simulink model "Lightning_McSeas_Dashboard_Copy"  (R2021b)
settings: Solver=VariableStepAuto  StartTime=0.0  StopTime=inf  RelTol=1e-3
undefined symbols (not defined in the file): canChannel
libraries: canmsglib x15, canlib x11
(part 2 of 2)

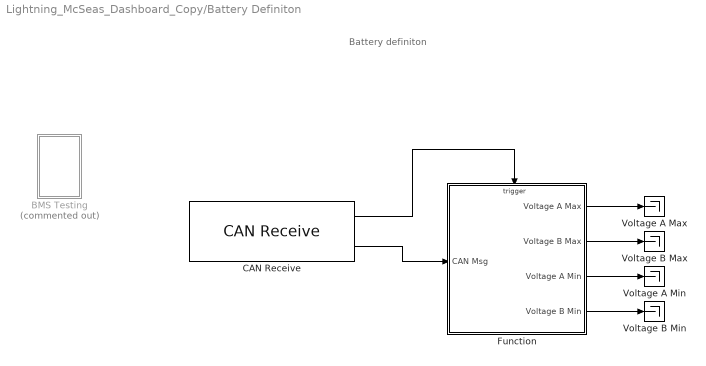
== system Lightning_McSeas_Dashboard_Copy/Battery Definiton ==
  note: Battery definiton
  BMS Testing : Subsystem  Commented=on
  CAN Receive : canlib/CAN Receive  BlockHandle=5.0006  Device=MathWorks Virtual 1 (Channel 1)  DeviceMenu=MathWorks Virtual 1 (Channel 1)  ObjConstructor=canChannel('MathWorks', 'Virtual 1', 1)  EnableStandardIDsFilter=off  StdIDsCombo=Allow all  StandardIDs=1536  EnableExtendedIDsFilter=off  ExtIDsCombo=Allow all  ExtendedIDs=0  SampleTime=0.1  MsgsPerTimestep=all  InternalFilterUpdateStatus=on  BusOutput=off
      settings: SourceProductBaseCode=VN
  Function : Subsystem  TreatAsAtomicUnit=on
  Voltage A Max : Terminator
  Voltage A Min : Terminator
  Voltage B Max : Terminator
  Voltage B Min : Terminator
  wires:
  CAN Receive/2 -> Function/1(CAN Msg)
  Function/1(Voltage A Max) -> Voltage A Max/1
  CAN Receive/1 -> Function/Trigger
  Function/2(Voltage B Max) -> Voltage B Max/1
  Function/3(Voltage A Min) -> Voltage A Min/1
  Function/4(Voltage B Min) -> Voltage B Min/1

== system Lightning_McSeas_Dashboard_Copy/GPS Definintion ==
  note: GPS definiton
  CAN Receive : canlib/CAN Receive  BlockHandle=24.0006  Device=MathWorks Virtual 1 (Channel 1)  DeviceMenu=MathWorks Virtual 1 (Channel 1)  ObjConstructor=canChannel('MathWorks', 'Virtual 1', 1)  EnableStandardIDsFilter=off  StdIDsCombo=Allow all  StandardIDs=1536  EnableExtendedIDsFilter=off  ExtIDsCombo=Allow all  ExtendedIDs=0  SampleTime=0.1  MsgsPerTimestep=all  InternalFilterUpdateStatus=on  BusOutput=off
      settings: SourceProductBaseCode=VN
  GPS Function : Subsystem  TreatAsAtomicUnit=on
  Speed : Terminator
  wires:
  CAN Receive/2 -> GPS Function/1(CAN Msg)
  GPS Function/1(Speed) -> Speed/1
  CAN Receive/1 -> GPS Function/Trigger

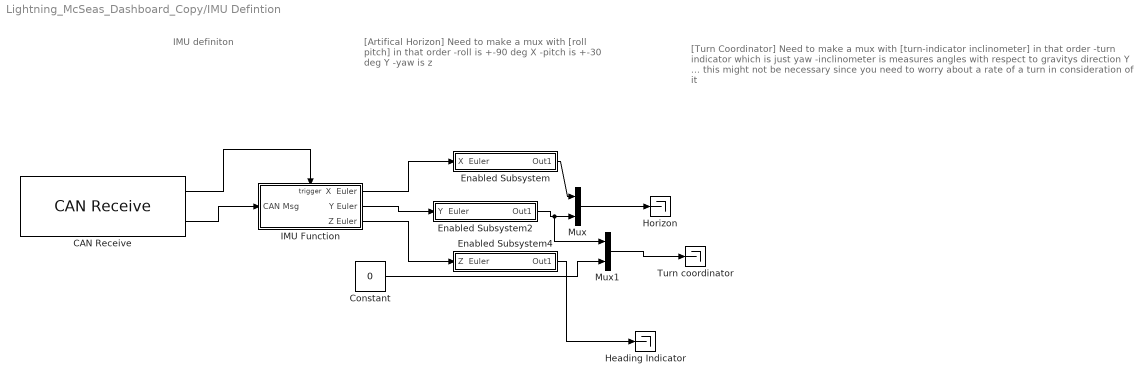
== system Lightning_McSeas_Dashboard_Copy/IMU Defintion ==
  note: [Turn Coordinator]
      | Need to make a mux with [turn-indicator inclinometer] in that order
      | -turn indicator which is just yaw
      |
      | -inclinometer is measures angles with respect to gravitys direction Y
      |
      | ... this might not be necessary since you need to worry about a rate of a turn in consideration of it
  note: [Artifical Horizon]
      | Need to make a mux with [roll pitch] in that order
      | -roll is +-90 deg X
      | -pitch is +-30 deg Y
      |
      | -yaw is z
  note: IMU definiton
  CAN Receive : canlib/CAN Receive  BlockHandle=40.0006  Device=MathWorks Virtual 1 (Channel 1)  DeviceMenu=MathWorks Virtual 1 (Channel 1)  ObjConstructor=canChannel('MathWorks', 'Virtual 1', 1)  EnableStandardIDsFilter=off  StdIDsCombo=Allow all  StandardIDs=1536  EnableExtendedIDsFilter=off  ExtIDsCombo=Allow all  ExtendedIDs=0  SampleTime=0.1  MsgsPerTimestep=all  InternalFilterUpdateStatus=on  BusOutput=off
      settings: SourceProductBaseCode=VN
  Constant : Constant  Value=0
  Enabled Subsystem : Subsystem  TreatAsAtomicUnit=on
  Enabled Subsystem2 : Subsystem  TreatAsAtomicUnit=on
  Enabled Subsystem4 : Subsystem  TreatAsAtomicUnit=on
  Heading Indicator : Terminator
  Horizon : Terminator
  IMU Function : Subsystem  TreatAsAtomicUnit=on
  Mux : Mux  Inputs=2
  Mux1 : Mux  Inputs=2
  Turn coordinator : Terminator
  wires:
  CAN Receive/2 -> IMU Function/1(CAN Msg)
  CAN Receive/1 -> IMU Function/Trigger
  Mux/1 -> Horizon/1
  Mux1/1 -> Turn coordinator/1
  Constant/1 -> Mux1/2
  IMU Function/1(X  Euler) -> Enabled Subsystem/1(X  Euler)
  Enabled Subsystem/1(Out1) -> Mux/1
  Enabled Subsystem2/1(Out1) -> Mux1/1, Mux/2
  IMU Function/2(Y Euler) -> Enabled Subsystem2/1(Y  Euler)
  IMU Function/3(Z Euler) -> Enabled Subsystem4/1(Z  Euler)
  Enabled Subsystem4/1(Out1) -> Heading Indicator/1

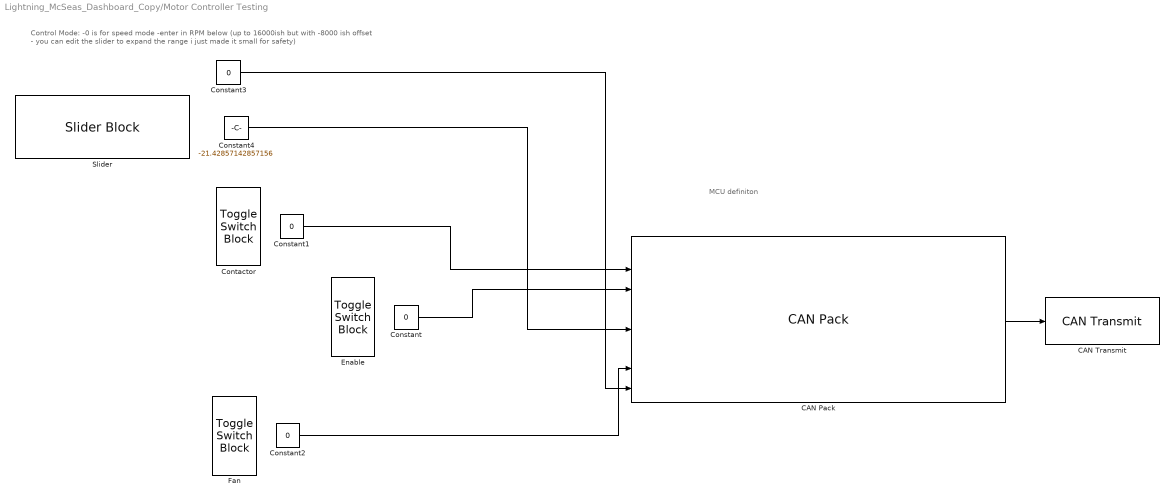
== system Lightning_McSeas_Dashboard_Copy/Motor Controller Testing ==
  note: Control Mode:
      | -0 is for speed mode
      | -enter in RPM below (up to 16000ish but with -8000 ish offset - you can edit the slider to expand the range i just made it small for safety)
  note: MCU definiton
  CAN Pack : canmsglib/CAN Pack  CANdbFile=C:\Users\jerod\OneDrive\Documents\School-Files\Boat_Team\GitHubFiles\dbc files\motor_controller.dbc  MsgList=Inv1_Command  MsgName=Inv1_Command  MsgIDType=Extended (29-bit identifier)  MsgIdentifier=218038727  MsgLength=8  Remote=off  ApplyMinMax=off  BusOutput=off  SignalInfo={ 'I1_CommandAcCurrent', '32', '16', 'LE', 'unsigned', 'Standard', '0', '0.05', '-1600', '-1600', '1676.75'; 'I1_CommandContact', '6', '2', 'LE', 'unsigned', 'Standard', '0', '1', '0', '-Inf', 'Inf'; 'I1_CommandEnable', '0', '2', 'LE', 'unsigned', 'Standard', '0', '1', '0', '-Inf', 'Inf'; 'I1_CommandFan', '8', '2', 'LE', 'unsigned', 'Standard', '0', '1', '0', '-Inf', 'Inf'; 'I1_CommandSpeed', '16', '16', 'LE', 'unsigned', 'Standard', '0', '0.25', '-8032.75', '-8032.75', '8351'; 'I1_CommandVoltage', '48', '16', 'LE', 'unsigned', 'Standard', '0', '0.05', '0', '0', '3276.75'; 'I1_EnableDebugMessages', '10', '2', 'LE', 'unsigned', 'Standard', '0', '1', '0', '-Inf', 'Inf'; 'I1_ReqControlMode', '2', '4', 'LE', 'unsigned', 'Standard', '0', '1', '0', '-Inf', 'Inf' }
      settings: SourceProductBaseCode=ME,XP,VN  DataFormat=CANdb specified signals
  CAN Transmit : canlib/CAN Transmit  BlockHandle=171.0006  Device=MathWorks Virtual 1 (Channel 1)  DeviceMenu=MathWorks Virtual 1 (Channel 1)  ObjConstructor=canChannel('MathWorks', 'Virtual 1', 1)  EnableEventTransmit=off  EnablePeriodicTransmit=off  MessagePeriod=1.000
      settings: SourceProductBaseCode=VN
  Constant{,1..3} (4 alike) : Constant  Value=0
  Constant4 : Constant  Value=-21.42857142857156
  Contactor : ToggleSwitchBlock
      settings: Values={{'Off', 'On'}, [0 1]}
  Enable : ToggleSwitchBlock
      settings: Values={{'Off', 'On'}, [0 1]}
  Fan : ToggleSwitchBlock
      settings: Values={{'Off', 'On'}, [0 1]}
  Slider : SliderBlock  ScaleMin=-8000  ScaleMax=8000
  wires:
  Constant1/1 -> CAN Pack/2
  Constant2/1 -> CAN Pack/7
  Constant3/1 -> CAN Pack/8
  CAN Pack/1 -> CAN Transmit/1
  Constant4/1 -> CAN Pack/5
  Constant/1 -> CAN Pack/3

== system Lightning_McSeas_Dashboard_Copy/Motor Definiton ==
  note: Need to add the information with all the rpm's, the temperatures
  note: Dashboard
  CAN Receive : canlib/CAN Receive  BlockHandle=190.0006  Device=MathWorks Virtual 1 (Channel 2)  DeviceMenu=MathWorks Virtual 1 (Channel 2)  ObjConstructor=canChannel('MathWorks', 'Virtual 1', 2)  EnableStandardIDsFilter=off  StdIDsCombo=Block all  StandardIDs=0  EnableExtendedIDsFilter=off  ExtIDsCombo=Allow all  ExtendedIDs=[50 100]  SampleTime=0.01  MsgsPerTimestep=all  InternalFilterUpdateStatus=on  BusOutput=on
      settings: SourceProductBaseCode=VN
  Dashboard ECU logic : Subsystem  TreatAsAtomicUnit=on
  RPM 1 : Terminator
  RPM 2 : Terminator
  wires:
  CAN Receive/1 -> Dashboard ECU logic/Trigger
  CAN Receive/2 -> Dashboard ECU logic/1(CAN message)
  Dashboard ECU logic/2(RPM 2) -> RPM 2/1
  Dashboard ECU logic/1(RPM 1) -> RPM 1/1

== system Lightning_McSeas_Dashboard_Copy/Test actuator ==
  CAN Pack : canmsglib/CAN Pack  CANdbFile=C:\Users\jerod\OneDrive\Documents\School-Files\Boat_Team\GitHubFiles\actuator_atmpt1.dbc  MsgList=actuator2  MsgName=actuator2  MsgIDType=Standard (11-bit identifier)  MsgIdentifier=31  MsgLength=2  Remote=off  ApplyMinMax=off  BusOutput=off  SignalInfo={ 'position_send2', '0', '16', 'LE', 'unsigned', 'Standard', '0', '1', '0', '-Inf', 'Inf' }
      settings: SourceProductBaseCode=ME,XP,VN  DataFormat=CANdb specified signals
  CAN Transmit : canlib/CAN Transmit  BlockHandle=249.0006  Device=MathWorks Virtual 1 (Channel 1)  DeviceMenu=MathWorks Virtual 1 (Channel 1)  ObjConstructor=canChannel('MathWorks', 'Virtual 1', 1)  EnableEventTransmit=off  EnablePeriodicTransmit=off  MessagePeriod=0.01
      settings: SourceProductBaseCode=VN
  Constant : Constant  Value=0
  Sine Wave : Sin  Commented=on  SineType=Sample based  Amplitude=32500  Bias=32500  Frequency=10  Samples=25  SampleTime=0.5
  Slider : SliderBlock  Commented=on  ScaleMax=65000
  wires:
  CAN Pack/1 -> CAN Transmit/1
  Constant/1 -> CAN Pack/1

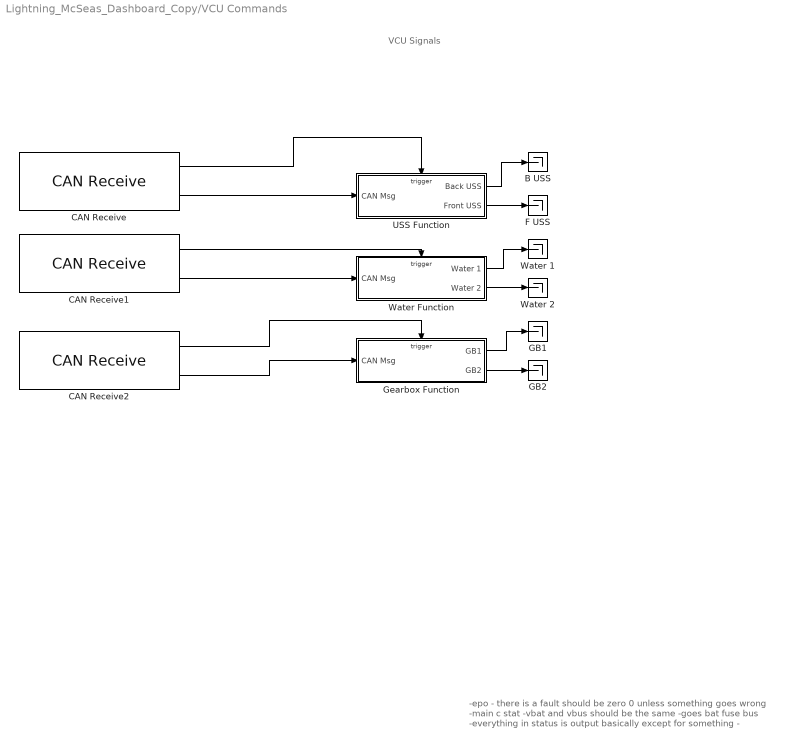
== system Lightning_McSeas_Dashboard_Copy/VCU Commands ==
  note: -epo - there is a fault should be zero 0 unless something goes wrong
      | -main c stat
      | -vbat and vbus should be the same
      | -goes bat fuse bus
      | -everything in status is output basically except for something
      | -
  note: VCU Signals
  B USS : Terminator
  CAN Receive : canlib/CAN Receive  BlockHandle=259.0006  Device=MathWorks Virtual 1 (Channel 1)  DeviceMenu=MathWorks Virtual 1 (Channel 1)  ObjConstructor=canChannel('MathWorks', 'Virtual 1', 1)  EnableStandardIDsFilter=off  StdIDsCombo=Allow all  StandardIDs=1536  EnableExtendedIDsFilter=off  ExtIDsCombo=Allow all  ExtendedIDs=0  SampleTime=0.1  MsgsPerTimestep=all  InternalFilterUpdateStatus=on  BusOutput=off
      settings: SourceProductBaseCode=VN
  CAN Receive1 : canlib/CAN Receive  BlockHandle=260.0006  Device=MathWorks Virtual 1 (Channel 1)  DeviceMenu=MathWorks Virtual 1 (Channel 1)  ObjConstructor=canChannel('MathWorks', 'Virtual 1', 1)  EnableStandardIDsFilter=off  StdIDsCombo=Allow all  StandardIDs=1536  EnableExtendedIDsFilter=off  ExtIDsCombo=Allow all  ExtendedIDs=0  SampleTime=0.1  MsgsPerTimestep=all  InternalFilterUpdateStatus=on  BusOutput=off
      settings: SourceProductBaseCode=VN
  CAN Receive2 : canlib/CAN Receive  BlockHandle=261.0006  Device=MathWorks Virtual 1 (Channel 1)  DeviceMenu=MathWorks Virtual 1 (Channel 1)  ObjConstructor=canChannel('MathWorks', 'Virtual 1', 1)  EnableStandardIDsFilter=off  StdIDsCombo=Allow all  StandardIDs=1536  EnableExtendedIDsFilter=off  ExtIDsCombo=Allow all  ExtendedIDs=0  SampleTime=0.1  MsgsPerTimestep=all  InternalFilterUpdateStatus=on  BusOutput=off
      settings: SourceProductBaseCode=VN
  F USS : Terminator
  GB1 : Terminator
  GB2 : Terminator
  Gearbox Function : Subsystem  TreatAsAtomicUnit=on
  USS Function : Subsystem  TreatAsAtomicUnit=on
  Water 1 : Terminator
  Water 2 : Terminator
  Water Function : Subsystem  TreatAsAtomicUnit=on
  wires:
  CAN Receive/2 -> USS Function/1(CAN Msg)
  CAN Receive/1 -> USS Function/Trigger
  USS Function/1(Back USS) -> B USS/1
  USS Function/2(Front USS) -> F USS/1
  Water Function/1(Water 1) -> Water 1/1
  Water Function/2(Water 2) -> Water 2/1
  CAN Receive1/2 -> Water Function/1(CAN Msg)
  CAN Receive1/1 -> Water Function/Trigger
  CAN Receive2/1 -> Gearbox Function/Trigger
  Gearbox Function/1(GB1) -> GB1/1
  Gearbox Function/2(GB2) -> GB2/1
  CAN Receive2/2 -> Gearbox Function/1(CAN Msg)

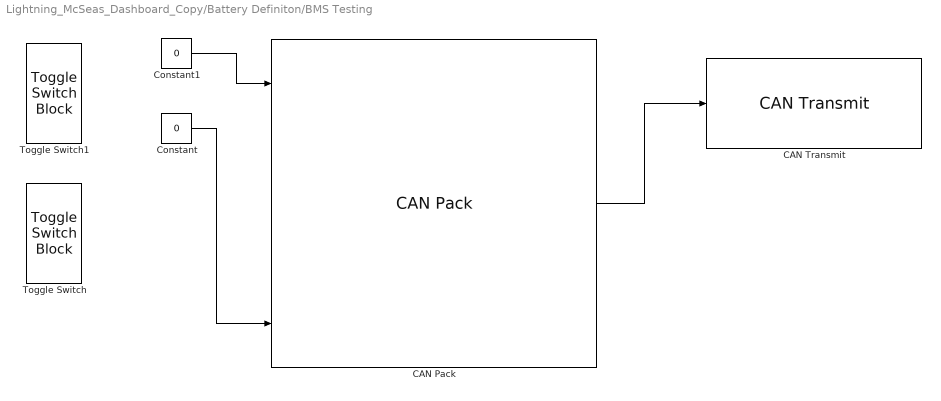
== system Lightning_McSeas_Dashboard_Copy/Battery Definiton/BMS Testing ==
  CAN Pack : canmsglib/CAN Pack  CANdbFile=C:\Users\jerod\OneDrive\Documents\School-Files\Boat_Team\GitHubFiles\BCM_VehBus_StdInterface.dbc  MsgList=BCM_Request  MsgName=BCM_Request  MsgIDType=Standard (11-bit identifier)  MsgIdentifier=1024  MsgLength=4  Remote=off  ApplyMinMax=off  BusOutput=off  SignalInfo={'hsc_bcm_enable','0','1','BE','unsigned','Standard','0','1','0','0','1';'hsc_bcm_epo','1','1','BE','unsigned','Standard','0','1','0','0','1';'hsc_bcm_leakage_ena','3','1','BE','unsigned','Standard','0','1','0','0','1';'hsc_bcm_mainc_close','2','1','BE','unsigned','Standard','0','1','0','0','1'}
      settings: SourceProductBaseCode=ME,XP,VN  DataFormat=CANdb specified signals
  CAN Transmit : canlib/CAN Transmit  BlockHandle=262.0006  Device=MathWorks Virtual 1 (Channel 1)  DeviceMenu=MathWorks Virtual 1 (Channel 1)  ObjConstructor=canChannel('MathWorks', 'Virtual 1', 1)  EnableEventTransmit=off  EnablePeriodicTransmit=off  MessagePeriod=1.000
      settings: SourceProductBaseCode=VN
  Constant : Constant  Value=0
  Constant1 : Constant  Value=0
  Toggle Switch : ToggleSwitchBlock
      settings: Values={{'Off', 'On'}, [0 1]}
  Toggle Switch1 : ToggleSwitchBlock
      settings: Values={{'Off', 'On'}, [0 1]}
  wires:
  CAN Pack/1 -> CAN Transmit/1
  Constant/1 -> CAN Pack/4
  Constant1/1 -> CAN Pack/1
  ? -> CAN Pack/2
  ? -> CAN Pack/3

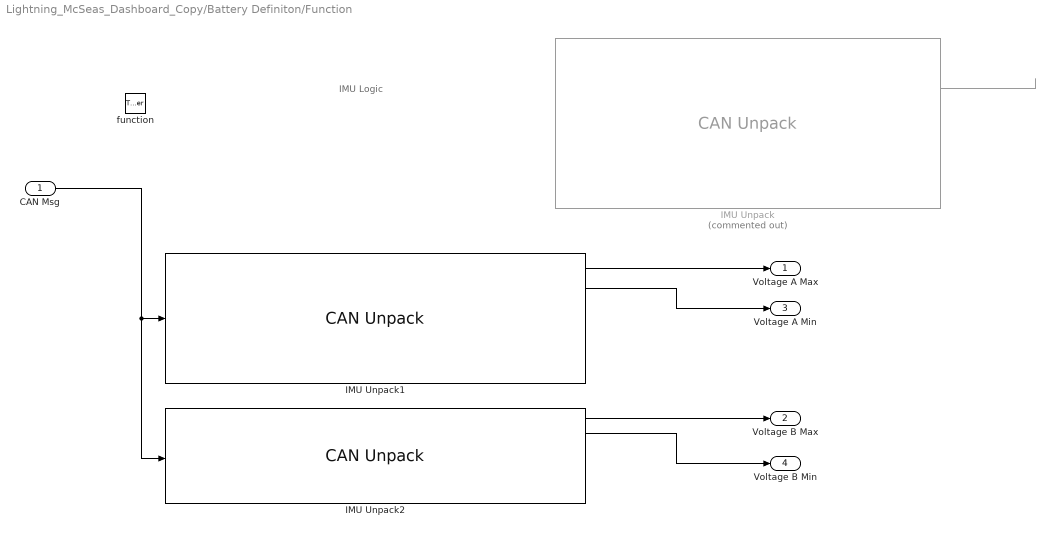
== system Lightning_McSeas_Dashboard_Copy/Battery Definiton/Function ==
  note: IMU Logic
  CAN Msg : Inport
  function : TriggerPort  TriggerType=function-call  VariantControl=(inherit)
  IMU Unpack : canmsglib/CAN Unpack  Commented=on  CANdbFile=C:\Users\jerod\OneDrive\Documents\School-Files\Boat_Team\GitHubFiles\dbc files\BCM_VehBus_StdInterface.dbc  MsgList=BCM_Status  MsgName=BCM_Status  MsgIDType=Standard (11-bit identifier)  MsgIdentifier=1040  MsgLength=8  SignalInfo={'bcm_alarm','14','2','BE','unsigned','Standard','0','1','0','0','3';'bcm_balancing','25','1','BE','unsigned','Standard','0','1','0','0','1';'bcm_cpwr_cmd','12','1','BE','unsigned','Standard','0','1','0','0','1';'bcm_cpwr_mon','13','1','BE','unsigned','Standard','0','1','0','0','1';'bcm_eeprom_wip','26','1','BE','unsigned','Standard','0','1','0','0','1';'bcm_epo','1','1','BE','unsigned','Standard','0','1','0','0','1';'bcm_fault_mon','27','1','BE','unsigned','Standard','0','1','0','0','1';'bcm_gfd','16','12','BE','unsigned','Standard','0','0.25','0','0','1000';'bcm_hvil_mon','3','1','BE','unsigned','Standard','0','1','0','0','1';'bcm_i_csm','40','16','BE','unsigned','Standard','0','0.025','-1000','-1000','500';'bcm_lvbat','56','8','BE','unsigned','Standard','0','0.2','0','0','51';'bcm_mainc_stat','4','2','BE','unsigned','Standard','0','1','0','0','2';'bcm_mainc_step','28','4','BE','unsigned','Standard','0','1','0','0','15';'bcm_mod_ena','7','1','BE','unsigned','Standard','0','1','0','0','1';'bcm_on_plug','2','1','BE','unsigned','Standard','0','1','0','0','1';'bcm_ready','0','1','BE','unsigned','Standard','0','1','0','0','1';'bcm_vbus_neg','48','8','BE','unsigned','Standard','0','1','-128','-128','127';'bcm_veh_mon','6','1','BE','unsigned','Standard','0','1','0','0','1'}  IDPort=off  TimestampPort=off  ErrorPort=off  RemotePort=off  LengthPort=off  StatusPort=off  ApplyMinMax=off
      settings: SourceProductBaseCode=ME,XP,VN  DataFormat=CANdb specified signals
  IMU Unpack1 : canmsglib/CAN Unpack  CANdbFile=C:\Users\jerod\OneDrive\Documents\School-Files\Boat_Team\GitHubFiles\dbc files\BCM_VehBus_StdInterface.dbc  MsgList=BCM_Meas_A  MsgName=BCM_Meas_A  MsgIDType=Standard (11-bit identifier)  MsgIdentifier=1072  MsgLength=8  SignalInfo={'bcm_cell_vmax_a','52','12','BE','unsigned','Standard','0','0.002','0','0','5';'bcm_cell_vmin_a','56','12','BE','unsigned','Standard','0','0.002','0','0','5';'bcm_i_lem_a','8','16','BE','unsigned','Standard','0','0.025','-1000','-1000','500';'bcm_vbat_a','16','8','BE','unsigned','Standard','0','0.5','0','0','125';'bcm_vbus_a','32','8','BE','unsigned','Standard','0','0.5','0','0','125';'bcm_vfuse_a','24','8','BE','unsigned','Standard','0','0.5','0','0','125'}  IDPort=off  TimestampPort=off  ErrorPort=off  RemotePort=off  LengthPort=off  StatusPort=off  ApplyMinMax=off
      settings: SourceProductBaseCode=ME,XP,VN  DataFormat=CANdb specified signals
  IMU Unpack2 : canmsglib/CAN Unpack  CANdbFile=C:\Users\jerod\OneDrive\Documents\School-Files\Boat_Team\GitHubFiles\dbc files\BCM_VehBus_StdInterface.dbc  MsgList=BCM_Meas_B  MsgName=BCM_Meas_B  MsgIDType=Standard (11-bit identifier)  MsgIdentifier=1073  MsgLength=8  SignalInfo={ 'bcm_cell_vmax_b', '52', '12', 'BE', 'unsigned', 'Standard', '0', '0.002', '0', '0', '5'; 'bcm_cell_vmin_b', '56', '12', 'BE', 'unsigned', 'Standard', '0', '0.002', '0', '0', '5'; 'bcm_i_lem_b', '8', '16', 'BE', 'unsigned', 'Standard', '0', '0.025', '-1000', '-1000', '500'; 'bcm_vbat_b', '16', '8', 'BE', 'unsigned', 'Standard', '0', '0.5', '0', '0', '125'; 'bcm_vbus_b', '32', '8', 'BE', 'unsigned', 'Standard', '0', '0.5', '0', '0', '125'; 'bcm_vfuse_b', '24', '8', 'BE', 'unsigned', 'Standard', '0', '0.5', '0', '0', '125' }  IDPort=off  TimestampPort=off  ErrorPort=off  RemotePort=off  LengthPort=off  StatusPort=off  ApplyMinMax=off
      settings: SourceProductBaseCode=ME,XP,VN  DataFormat=CANdb specified signals
  Voltage A Max : Outport
  Voltage B Max : Outport  Port=2
  Voltage A Min : Outport  Port=3
  Voltage B Min : Outport  Port=4
  wires:
  IMU Unpack1/1 -> Voltage A Max/1
  CAN Msg/1 -> IMU Unpack2/1, IMU Unpack1/1
  IMU Unpack2/1 -> Voltage B Max/1
  IMU Unpack/6 -> ?
  IMU Unpack1/2 -> Voltage A Min/1
  IMU Unpack2/2 -> Voltage B Min/1

== system Lightning_McSeas_Dashboard_Copy/GPS Definintion/GPS Function ==
  note: IMU Logic
  CAN Msg : Inport
  function : TriggerPort  TriggerType=function-call  VariantControl=(inherit)
  IMU Unpack : canmsglib/CAN Unpack  CANdbFile=C:\Users\jerod\OneDrive\Documents\School-Files\Boat_Team\GitHubFiles\PCAN-GPS_Symbols.dbc  MsgList=GPS_CourseSpeed  MsgName=GPS_CourseSpeed  MsgIDType=Standard (11-bit identifier)  MsgIdentifier=1569  MsgLength=8  SignalInfo={'GPS_Course','0','32','LE','single','Standard','0','1','0','-3.4e+38','3.4e+38';'GPS_Speed','32','32','LE','single','Standard','0','1','0','-3.4e+38','3.4e+38'}  IDPort=off  TimestampPort=off  ErrorPort=off  RemotePort=off  LengthPort=off  StatusPort=off  ApplyMinMax=off
      settings: SourceProductBaseCode=ME,XP,VN  DataFormat=CANdb specified signals
  Speed : Outport
  wires:
  IMU Unpack/2 -> Speed/1
  CAN Msg/1 -> IMU Unpack/1

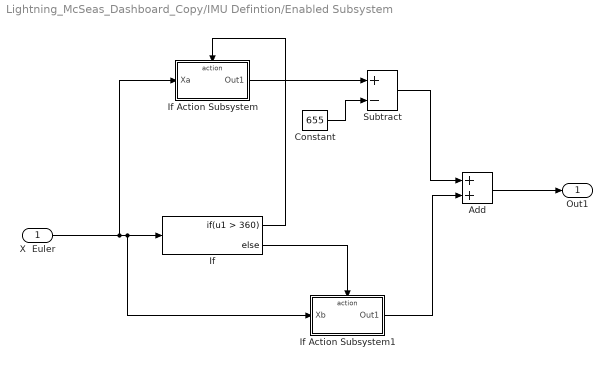
== system Lightning_McSeas_Dashboard_Copy/IMU Defintion/Enabled Subsystem ==
  X  Euler : Inport
  Add : Sum
  Constant : Constant  Value=655
  If : If  IfExpression=u1 > 360
  If Action Subsystem : Subsystem  TreatAsAtomicUnit=on
  If Action Subsystem1 : Subsystem  TreatAsAtomicUnit=on
  Subtract : Sum  Inputs=+-
  Out1 : Outport
  wires:
  If/1 -> If Action Subsystem/Action
  Constant/1 -> Subtract/2
  If/2 -> If Action Subsystem1/Action
  Add/1 -> Out1/1
  Subtract/1 -> Add/1
  X  Euler/1 -> If Action Subsystem/1(Xa), If Action Subsystem1/1(Xb), If/1
  If Action Subsystem/1(Out1) -> Subtract/1
  If Action Subsystem1/1(Out1) -> Add/2

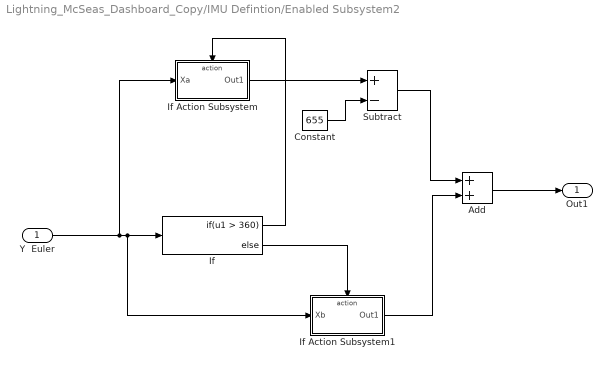
== system Lightning_McSeas_Dashboard_Copy/IMU Defintion/Enabled Subsystem2 ==
  Y  Euler : Inport
  Add : Sum
  Constant : Constant  Value=655
  If : If  IfExpression=u1 > 360
  If Action Subsystem : Subsystem  TreatAsAtomicUnit=on
  If Action Subsystem1 : Subsystem  TreatAsAtomicUnit=on
  Subtract : Sum  Inputs=+-
  Out1 : Outport
  wires:
  If/1 -> If Action Subsystem/Action
  Constant/1 -> Subtract/2
  If/2 -> If Action Subsystem1/Action
  Add/1 -> Out1/1
  Subtract/1 -> Add/1
  Y  Euler/1 -> If Action Subsystem/1(Xa), If Action Subsystem1/1(Xb), If/1
  If Action Subsystem/1(Out1) -> Subtract/1
  If Action Subsystem1/1(Out1) -> Add/2

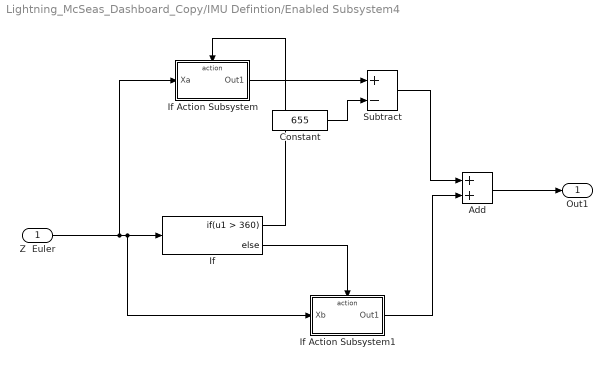
== system Lightning_McSeas_Dashboard_Copy/IMU Defintion/Enabled Subsystem4 ==
  Z  Euler : Inport
  Add : Sum
  Constant : Constant  Value=655
  If : If  IfExpression=u1 > 360
  If Action Subsystem : Subsystem  TreatAsAtomicUnit=on
  If Action Subsystem1 : Subsystem  TreatAsAtomicUnit=on
  Subtract : Sum  Inputs=+-
  Out1 : Outport
  wires:
  If/1 -> If Action Subsystem/Action
  Constant/1 -> Subtract/2
  If/2 -> If Action Subsystem1/Action
  Add/1 -> Out1/1
  Subtract/1 -> Add/1
  Z  Euler/1 -> If Action Subsystem/1(Xa), If Action Subsystem1/1(Xb), If/1
  If Action Subsystem/1(Out1) -> Subtract/1
  If Action Subsystem1/1(Out1) -> Add/2

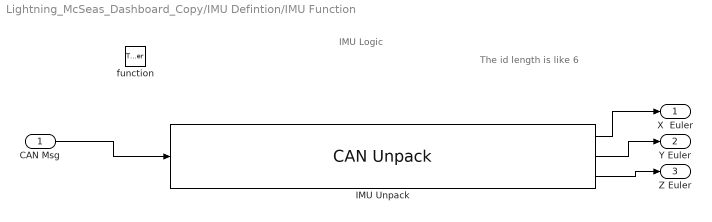
== system Lightning_McSeas_Dashboard_Copy/IMU Defintion/IMU Function ==
  note: The id length is like 6
  note: IMU Logic
  CAN Msg : Inport
  function : TriggerPort  TriggerType=function-call  VariantControl=(inherit)
  IMU Unpack : canmsglib/CAN Unpack  CANdbFile=C:\Users\jerod\OneDrive\Documents\School-Files\Boat_Team\GitHubFiles\LPMS_IMU.dbc  MsgList=IMU_Euler_Angles  MsgName=IMU_Euler_Angles  MsgIDType=Standard (11-bit identifier)  MsgIdentifier=1301  MsgLength=6  SignalInfo={ 'Euler_X', '0', '16', 'LE', 'unsigned', 'Standard', '0', '0.01', '0', '-180', '180'; 'Euler_Y', '16', '16', 'LE', 'unsigned', 'Standard', '0', '0.01', '0', '-90', '90'; 'Euler_Z', '32', '16', 'LE', 'unsigned', 'Standard', '0', '0.01', '0', '-180', '180' }  IDPort=off  TimestampPort=off  ErrorPort=off  RemotePort=off  LengthPort=off  StatusPort=off  ApplyMinMax=off
      settings: SourceProductBaseCode=ME,XP,VN
  X  Euler : Outport
  Y Euler : Outport  Port=2
  Z Euler : Outport  Port=3
  wires:
  IMU Unpack/3 -> Z Euler/1
  IMU Unpack/1 -> X  Euler/1
  IMU Unpack/2 -> Y Euler/1
  CAN Msg/1 -> IMU Unpack/1

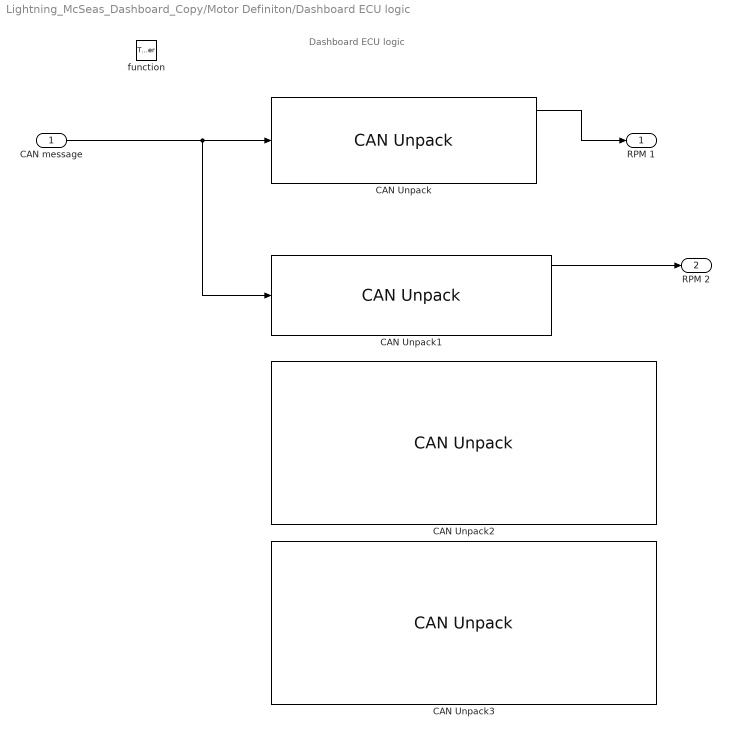
== system Lightning_McSeas_Dashboard_Copy/Motor Definiton/Dashboard ECU logic ==
  note: Dashboard ECU logic
  CAN message : Inport
  function : TriggerPort  TriggerType=function-call  VariantControl=Variant
  CAN Unpack : canmsglib/CAN Unpack  CANdbFile=C:\Users\jerod\OneDrive\Documents\School-Files\Boat_Team\GitHubFiles\dbc files\motor_controller.dbc  MsgList=Inv1_Actual  MsgName=Inv1_Actual  MsgIDType=Extended (29-bit identifier)  MsgIdentifier=218039240  MsgLength=8  SignalInfo={ 'I1_ActualSpeed', '0', '16', 'LE', 'unsigned', 'Standard', '0', '0.25', '-8032.75', '-8032.75', '8351'; 'I1_DcBusCurrent', '48', '16', 'LE', 'unsigned', 'Standard', '0', '0.05', '-1600', '-1600', '1676.75'; 'I1_DcBusVoltage', '32', '16', 'LE', 'unsigned', 'Standard', '0', '0.05', '0', '0', '3276.75'; 'I1_RmsMotorCurrent', '16', '16', 'LE', 'unsigned', 'Standard', '0', '0.05', '-1600', '-1600', '1676.75' }  IDPort=off  TimestampPort=off  ErrorPort=off  RemotePort=off  LengthPort=off  StatusPort=off  ApplyMinMax=off
      settings: SourceProductBaseCode=ME,XP,VN  DataFormat=CANdb specified signals
  CAN Unpack1 : canmsglib/CAN Unpack  CANdbFile=C:\Users\jerod\OneDrive\Documents\School-Files\Boat_Team\GitHubFiles\dbc files\motor_controller.dbc  MsgList=Inv2_Actual  MsgName=Inv2_Actual  MsgIDType=Extended (29-bit identifier)  MsgIdentifier=218043336  MsgLength=8  SignalInfo={ 'I2_ActualSpeed', '0', '16', 'LE', 'unsigned', 'Standard', '0', '0.25', '-8032.75', '-8032.75', '8351'; 'I2_DcBusCurrent', '48', '16', 'LE', 'unsigned', 'Standard', '0', '0.05', '-1600', '-1600', '1676.75'; 'I2_DcBusVoltage', '32', '16', 'LE', 'unsigned', 'Standard', '0', '0.05', '0', '0', '3276.75'; 'I2_RmsMotorCurrent', '16', '16', 'LE', 'unsigned', 'Standard', '0', '0.05', '-1600', '-1600', '1676.75' }  IDPort=off  TimestampPort=off  ErrorPort=off  RemotePort=off  LengthPort=off  StatusPort=off  ApplyMinMax=off
      settings: SourceProductBaseCode=ME,XP,VN  DataFormat=CANdb specified signals
  CAN Unpack2 : canmsglib/CAN Unpack  CANdbFile=C:\Users\jerod\OneDrive\Documents\School-Files\Boat_Team\GitHubFiles\dbc files\motor_controller.dbc  MsgList=Inv1_Status  MsgName=Inv1_Status  MsgIDType=Extended (29-bit identifier)  MsgIdentifier=218039496  MsgLength=8  SignalInfo={ 'I1_ActualControlMode', '4', '4', 'LE', 'unsigned', 'Standard', '0', '1', '0', '-Inf', 'Inf'; 'I1_ActualStatus', '0', '4', 'LE', 'unsigned', 'Standard', '0', '1', '0', '-Inf', 'Inf'; 'I1_DcBusDerate', '22', '2', 'LE', 'unsigned', 'Standard', '0', '1', '0', '-Inf', 'Inf'; 'I1_DriveTempDerate', '16', '2', 'LE', 'unsigned', 'Standard', '0', '1', '0', '-Inf', 'Inf'; 'I1_DriveTemperature', '40', '8', 'LE', 'unsigned', 'Standard', '0', '1', '-40', '-40', '215'; 'I1_ErrorActive', '8', '2', 'LE', 'unsigned', 'Standard', '0', '1', '0', '-Inf', 'Inf'; 'I1_MotorTempDerate', '18', '2', 'LE', 'unsigned', 'Standard', '0', '1', '0', '-Inf', 'Inf'; 'I1_MotorTemperature', '32', '8', 'LE', 'unsigned', 'Standard', '0', '1', '-40', '-40', '215'; 'I1_Saturated', '10', '2', 'LE', 'unsigned', 'Standard', '0', '1', '0', '-Inf', 'Inf'; 'I1_SpeedDerate', '20', '2', 'LE', 'unsigned', 'Standard', '0', '1', '0', '-Inf', 'Inf' }  IDPort=off  TimestampPort=off  ErrorPort=off  RemotePort=off  LengthPort=off  StatusPort=off  ApplyMinMax=off
      settings: SourceProductBaseCode=ME,XP,VN  DataFormat=CANdb specified signals
  CAN Unpack3 : canmsglib/CAN Unpack  CANdbFile=C:\Users\jerod\OneDrive\Documents\School-Files\Boat_Team\GitHubFiles\dbc files\motor_controller.dbc  MsgList=Inv1_Status  MsgName=Inv1_Status  MsgIDType=Extended (29-bit identifier)  MsgIdentifier=218039496  MsgLength=8  SignalInfo={'I1_ActualControlMode','4','4','LE','unsigned','Standard','0','1','0','-Inf','Inf';'I1_ActualStatus','0','4','LE','unsigned','Standard','0','1','0','-Inf','Inf';'I1_DcBusDerate','22','2','LE','unsigned','Standard','0','1','0','-Inf','Inf';'I1_DriveTempDerate','16','2','LE','unsigned','Standard','0','1','0','-Inf','Inf';'I1_DriveTemperature','40','8','LE','unsigned','Standard','0','1','-40','-40','215';'I1_ErrorActive','8','2','LE','unsigned','Standard','0','1','0','-Inf','Inf';'I1_MotorTempDerate','18','2','LE','unsigned','Standard','0','1','0','-Inf','Inf';'I1_MotorTemperature','32','8','LE','unsigned','Standard','0','1','-40','-40','215';'I1_Saturated','10','2','LE','unsigned','Standard','0','1','0','-Inf','Inf';'I1_SpeedDerate','20','2','LE','unsigned','Standard','0','1','0','-Inf','Inf'}  IDPort=off  TimestampPort=off  ErrorPort=off  RemotePort=off  LengthPort=off  StatusPort=off  ApplyMinMax=off
      settings: SourceProductBaseCode=ME,XP,VN  DataFormat=CANdb specified signals
  RPM 1 : Outport  VectorParamsAs1DForOutWhenUnconnected=off
  RPM 2 : Outport  Port=2  VectorParamsAs1DForOutWhenUnconnected=off
  wires:
  CAN message/1 -> CAN Unpack1/1, CAN Unpack/1
  CAN Unpack/1 -> RPM 1/1
  CAN Unpack1/1 -> RPM 2/1

== system Lightning_McSeas_Dashboard_Copy/VCU Commands/Gearbox Function ==
  note: IMU Logic
  CAN Msg : Inport
  function : TriggerPort  TriggerType=function-call  VariantControl=(inherit)
  IMU Unpack : canmsglib/CAN Unpack  CANdbFile=C:\Users\jerod\OneDrive\Documents\School-Files\Boat_Team\GitHubFiles\LPMS_IMU.dbc  MsgList=Gearbox_Temps  MsgName=Gearbox_Temps  MsgIDType=Standard (11-bit identifier)  MsgIdentifier=1307  MsgLength=8  SignalInfo={'Gearbox1','0','16','LE','unsigned','Standard','0','1','0','-Inf','Inf';'Gearbox2','16','16','LE','unsigned','Standard','0','1','0','-Inf','Inf'}  IDPort=off  TimestampPort=off  ErrorPort=off  RemotePort=off  LengthPort=off  StatusPort=off  ApplyMinMax=off
      settings: SourceProductBaseCode=ME,XP,VN  DataFormat=CANdb specified signals
  GB1 : Outport
  GB2 : Outport  Port=2
  wires:
  IMU Unpack/1 -> GB1/1
  IMU Unpack/2 -> GB2/1
  CAN Msg/1 -> IMU Unpack/1

== system Lightning_McSeas_Dashboard_Copy/VCU Commands/USS Function ==
  note: IMU Logic
  CAN Msg : Inport
  function : TriggerPort  TriggerType=function-call  VariantControl=(inherit)
  IMU Unpack : canmsglib/CAN Unpack  CANdbFile=C:\Users\jerod\OneDrive\Documents\School-Files\Boat_Team\LPMS_IMU.dbc  MsgList=UltraSonic_Voltage  MsgName=UltraSonic_Voltage  MsgIDType=Standard (11-bit identifier)  MsgIdentifier=1  MsgLength=8  SignalInfo={'BackSensorReading','16','1','LE','unsigned','Standard','0','1','0','-Inf','Inf';'FrontSensorReading','0','16','LE','unsigned','Standard','0','1','0','-Inf','Inf'}  IDPort=off  TimestampPort=off  ErrorPort=off  RemotePort=off  LengthPort=off  StatusPort=off  ApplyMinMax=off
      settings: SourceProductBaseCode=ME,XP,VN  DataFormat=CANdb specified signals
  Back USS : Outport
  Front USS : Outport  Port=2
  wires:
  IMU Unpack/1 -> Back USS/1
  IMU Unpack/2 -> Front USS/1
  CAN Msg/1 -> IMU Unpack/1

== system Lightning_McSeas_Dashboard_Copy/VCU Commands/Water Function ==
  note: IMU Logic
  CAN Msg : Inport
  function : TriggerPort  TriggerType=function-call  VariantControl=(inherit)
  IMU Unpack : canmsglib/CAN Unpack  CANdbFile=C:\Users\jerod\OneDrive\Documents\School-Files\Boat_Team\GitHubFiles\LPMS_IMU.dbc  MsgList=Water_Sensor_V_H  MsgName=Water_Sensor_V_H  MsgIDType=Standard (11-bit identifier)  MsgIdentifier=1306  MsgLength=8  SignalInfo={'Water_Sensor_1','0','1','LE','unsigned','Standard','0','1','0','-Inf','Inf';'Water_Sensor_2','1','1','LE','unsigned','Standard','0','1','0','-Inf','Inf'}  IDPort=off  TimestampPort=off  ErrorPort=off  RemotePort=off  LengthPort=off  StatusPort=off  ApplyMinMax=off
      settings: SourceProductBaseCode=ME,XP,VN  DataFormat=CANdb specified signals
  Water 1 : Outport
  Water 2 : Outport  Port=2
  wires:
  IMU Unpack/1 -> Water 1/1
  IMU Unpack/2 -> Water 2/1
  CAN Msg/1 -> IMU Unpack/1

== system Lightning_McSeas_Dashboard_Copy/IMU Defintion/Enabled Subsystem/If Action Subsystem ==
  Xa : Inport
  Action Port : ActionPort  ActionPortLabel=if(u1 > 360)
  Out1 : Outport
  wires:
  Xa/1 -> Out1/1

== system Lightning_McSeas_Dashboard_Copy/IMU Defintion/Enabled Subsystem/If Action Subsystem1 ==
  Xb : Inport
  Action Port : ActionPort  ActionPortLabel=else
  Out1 : Outport
  wires:
  Xb/1 -> Out1/1

== system Lightning_McSeas_Dashboard_Copy/IMU Defintion/Enabled Subsystem2/If Action Subsystem ==
  Xa : Inport
  Action Port : ActionPort  ActionPortLabel=if(u1 > 360)
  Out1 : Outport
  wires:
  Xa/1 -> Out1/1

== system Lightning_McSeas_Dashboard_Copy/IMU Defintion/Enabled Subsystem2/If Action Subsystem1 ==
  Xb : Inport
  Action Port : ActionPort  ActionPortLabel=else
  Out1 : Outport
  wires:
  Xb/1 -> Out1/1

== system Lightning_McSeas_Dashboard_Copy/IMU Defintion/Enabled Subsystem4/If Action Subsystem ==
  Xa : Inport
  Action Port : ActionPort  ActionPortLabel=if(u1 > 360)
  Out1 : Outport
  wires:
  Xa/1 -> Out1/1

== system Lightning_McSeas_Dashboard_Copy/IMU Defintion/Enabled Subsystem4/If Action Subsystem1 ==
  Xb : Inport
  Action Port : ActionPort  ActionPortLabel=else
  Out1 : Outport
  wires:
  Xb/1 -> Out1/1
